simulink model "window_discriminator_5_2016"  (Simulink 8.8)
settings: Solver=FixedStepAuto  StartTime=0.0  StopTime=197  RelTol=1e-3
model workspace (MAT data in the model file):
  dac_stop_max = 3
  threshold = [-50; -300]
  win_start = [0; 0]
  win_stop = [3; 3]
PreLoadFcn:
  | load('DAC_data_0.mat')
libraries: simulink x28, dspswit3 x2
settings Model: SuppressorTable=22 serialization::archive 11 0 6 0 0 0 0 0  LogicAnalyzerGraphicalSettings="{\"cursors\":{\"activeCursor\":3,\"lockedCursors\":[],\"startingCursor\":0,\"times\":[0,4.8,0.93912000000000018,0.71536000000000011]},\"global\":{\"color\":\"#ff0000\",\"radix\":\"binary\",\"spacing\":20},\"panels\":{\"height\":100,\"startingTrace\":0,\"traces\":[{\"signalId\":\"f8938369-8c5b-4d01-b24d-9cd3e4e46d98\",\"type\":\"wave\"},{\"signalId\":\"94a143c0-ec74-472f-a084-edb62442a186\",\"type\":\"wave\"},{\"signalId\":\"701b10aa-339e-45e1-9be0-5d4a727281ed\",\"type\":\"wave\"},{\"signalId\":\"013b7378-a8ba-49d0-af91-3fbd95361aac\",\"type\":\"wave\"},{\"signalId\":\"480a99f9-8d02-4e3a-b326-8ef0fd120828\",\"type\":\"wave\"},{\"signalId\":\"c0ccc7cd-eb1d-43ab-8d7f-fc260d9b67b0\",\"type\":\"wave\"},{\"signalId\":\"28e0c295-4c7e-4ad9-b928-034bfdabfe57\",\"type\":\"wave\"},{\"signalId\":\"c5377225-ef61-4e55-bb70-795e7293a3ed\",\"type\":\"wave\"},{\"signalId\":\"41701cb5-c102-4d46-8782-f91045dab3d0\",\"type\":\"wave\"},{\"signalId\":\"59c9867a-a6c4-4660-9624-649cf34ef1b0\",\"type\":\"wave\"}],\"yOffset\":0},\"timeAxis\":{\"pixelsPerSecond\":1.8481561822124021E+6},\"trigger\":{\"enabled\":false,\"mode\":\"once\",\"samples\":200,\"signals\":{},\"stages\":{\"conditions\":[],\"operator\":\"AND\"}}}"  Creator=stefanobuccelli  LastModifiedBy=stefanobuccelli  SimulationMode=accelerator
settings DataIOCC: LimitDataPoints=off  SaveFormat=Dataset  SignalLoggingSaveFormat=Dataset
settings OptimizationCC: LifeSpan=auto
settings DebuggingCC: UnderspecifiedInitializationDetection=Simplified  MergeDetectMultiDrivingBlocksExec=error  FcnCallInpInsideContextMsg=error  StateNameClashWarn=none  SFUnexpectedBacktrackingDiag=error  SFNoUnconditionalDefaultTransitionDiag=error  SFExecutionAtInitializationDiag=warning
settings HardwareCC: ProdBitPerPointer=64  ProdBitPerSizeT=64  ProdBitPerPtrDiffT=64  ProdLargestAtomicFloat=Float  ProdIntDivRoundTo=Zero  ProdEndianess=LittleEndian  ProdWordSize=64  ProdHWDeviceType=Intel->x86-64 (Windows64)
settings ModelReferenceCC: PropagateSignalLabelsOutOfModel=on
settings GRTTargetCC: TargetLangStandard=C99 (ISO)  GeneratePreprocessorConditionals=Use local settings  CombineOutputUpdateFcns=on  GRTInterface=off
settings ConfigComp: CovMetricSettings=dwe  CovHtmlReporting=off  CovSaveCumulativeToWorkspaceVar=off  CovSaveSingleToWorkspaceVar=off  CovExternalEMLEnable=on

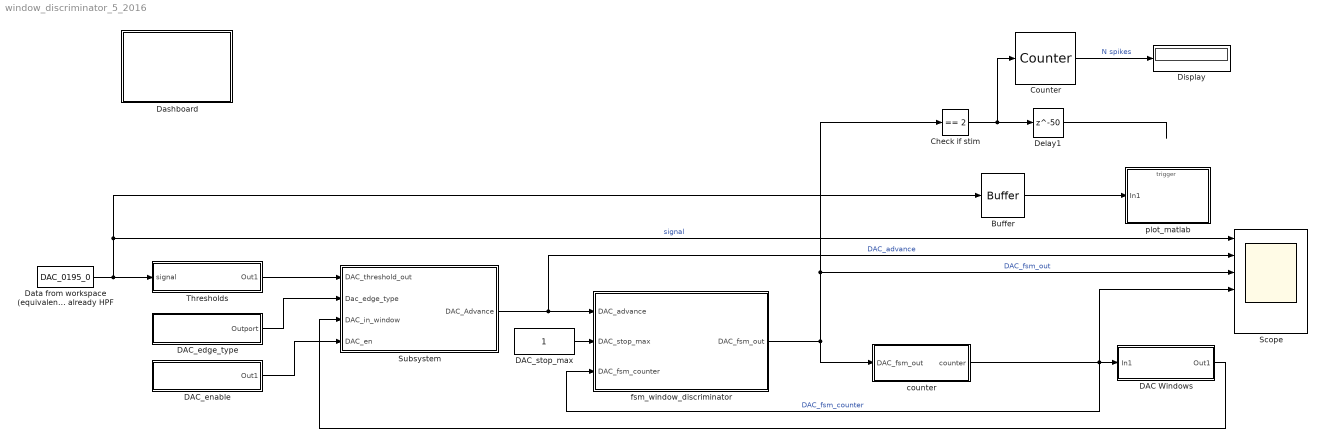
== system window_discriminator_5_2016 ==
  Buffer : Buffer  N=100  V=99  OutputFrames=off
  Check if stim : simulink/Logic and Bit Operations/Compare To Constant  relop===  const=2  OutDataTypeStr=boolean
  Counter : dspswit3/Counter  Direction=Up  CountEvent=Rising edge  CounterSize=User defined  MaxCount=1e6  InitialCount=0  Output=Count  HitValue=32  ResetInput=off  SamplesPerFrame=1  Ts=1  CntDtype=double  HitDtype=Logical
  DAC Windows : Subsystem
  DAC_edge_type : Subsystem
  DAC_enable : Subsystem
  DAC_stop_max : Constant  OutDataTypeStr=double
  Dashboard : Subsystem
  Data from workspace (equivalent  to the board_DAC_data the one already HPF : FromWorkspace  VariableName=DAC_0195_0  SampleTime=1/30000
  Delay1 : Delay  DelayLength=50
  Display : Display
  Scope : Scope  NumInputPorts=6
  Subsystem : Subsystem
  Thresholds : Subsystem
  counter : Subsystem
  fsm_window_discriminator : Stateflow chart  TreatAsAtomicUnit=on
  plot_matlab : Subsystem
  wires:
  fsm_window_discriminator/1(DAC_fsm_out) -> counter/1(DAC_fsm_out), Check if stim/1, Scope/3  "DAC_fsm_out"
  Data from workspace (equivalent  to the board_DAC_data the one already HPF/1 -> Buffer/1, Scope/1, Thresholds/1(signal)  "signal"
  Subsystem/1(DAC_Advance) -> Scope/2, fsm_window_discriminator/1(DAC_advance)  "DAC_advance"
  DAC_edge_type/1(Outport) -> Subsystem/2(Dac_edge_type)
  DAC_stop_max/1 -> fsm_window_discriminator/2(DAC_stop_max)
  Check if stim/1 -> Counter/1, Delay1/1
  Buffer/1 -> plot_matlab/1(In1)
  Delay1/1 -> ?
  DAC Windows/1(Out1) -> Subsystem/3(DAC_in_window)
  Thresholds/1(Out1) -> Subsystem/1(DAC_threshold_out)
  DAC_enable/1(Out1) -> Subsystem/4(DAC_en)
  counter/1(counter) -> fsm_window_discriminator/3(DAC_fsm_counter), DAC Windows/1(In1), Scope/4  "DAC_fsm_counter"
  Counter/1 -> Display/1  "N spikes"

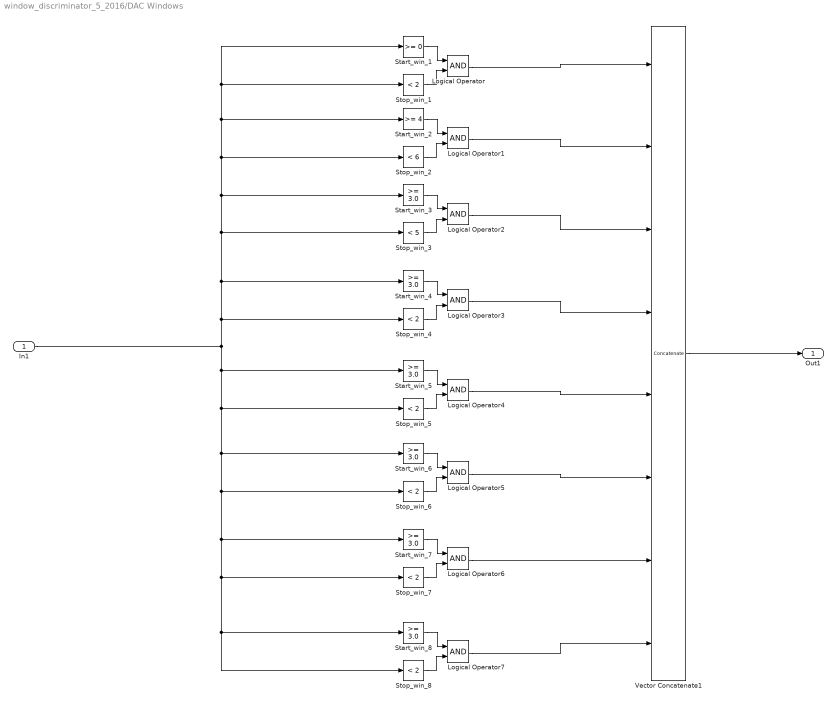
== system window_discriminator_5_2016/DAC Windows ==
  In1 : Inport
  Logical Operator{,1..7} (8 alike) : Logic  AllPortsSameDT=off  OutDataTypeStr=boolean
  Start_win_1 : simulink/Logic and Bit Operations/Compare To Constant  relop=>=  const=0  OutDataTypeStr=boolean
  Start_win_2 : simulink/Logic and Bit Operations/Compare To Constant  relop=>=  const=4  OutDataTypeStr=boolean
  Start_win_{3..8} (6 alike) : simulink/Logic and Bit Operations/Compare To Constant  relop=>=  const=3.0  OutDataTypeStr=boolean
  Stop_win_{1,4..8} (6 alike) : simulink/Logic and Bit Operations/Compare To Constant  relop=<  const=2  OutDataTypeStr=boolean
  Stop_win_2 : simulink/Logic and Bit Operations/Compare To Constant  relop=<  const=6  OutDataTypeStr=boolean
  Stop_win_3 : simulink/Logic and Bit Operations/Compare To Constant  relop=<  const=5  OutDataTypeStr=boolean
  Vector Concatenate1 : Concatenate  NumInputs=8
  Out1 : Outport
  wires:
  Vector Concatenate1/1 -> Out1/1
  Stop_win_1/1 -> Logical Operator/2
  Start_win_1/1 -> Logical Operator/1
  Logical Operator/1 -> Vector Concatenate1/1
  Logical Operator1/1 -> Vector Concatenate1/2
  Stop_win_2/1 -> Logical Operator1/2
  Start_win_2/1 -> Logical Operator1/1
  Stop_win_3/1 -> Logical Operator2/2
  Start_win_3/1 -> Logical Operator2/1
  Logical Operator2/1 -> Vector Concatenate1/3
  Start_win_4/1 -> Logical Operator3/1
  Stop_win_4/1 -> Logical Operator3/2
  Logical Operator3/1 -> Vector Concatenate1/4
  Stop_win_5/1 -> Logical Operator4/2
  Start_win_5/1 -> Logical Operator4/1
  Logical Operator4/1 -> Vector Concatenate1/5
  Start_win_6/1 -> Logical Operator5/1
  Logical Operator5/1 -> Vector Concatenate1/6
  Stop_win_6/1 -> Logical Operator5/2
  Stop_win_7/1 -> Logical Operator6/2
  Start_win_7/1 -> Logical Operator6/1
  Logical Operator6/1 -> Vector Concatenate1/7
  Stop_win_8/1 -> Logical Operator7/2
  Start_win_8/1 -> Logical Operator7/1
  Logical Operator7/1 -> Vector Concatenate1/8
  In1/1 -> Stop_win_5/1, Start_win_6/1, Stop_win_6/1, Start_win_7/1, Stop_win_7/1, Start_win_8/1, Stop_win_8/1, Start_win_5/1, Stop_win_4/1, Start_win_4/1, Stop_win_3/1, Start_win_3/1, Stop_win_2/1, Start_win_2/1, Stop_win_1/1, Start_win_1/1

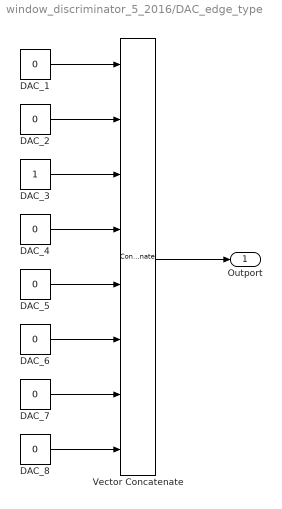
== system window_discriminator_5_2016/DAC_edge_type ==
  DAC_{1..2,4..8} (7 alike) : Constant  Value=0
  DAC_3 : Constant
  Vector Concatenate : Concatenate  NumInputs=8
  Outport : Outport
  wires:
  DAC_7/1 -> Vector Concatenate/7
  DAC_6/1 -> Vector Concatenate/6
  DAC_1/1 -> Vector Concatenate/1
  Vector Concatenate/1 -> Outport/1
  DAC_5/1 -> Vector Concatenate/5
  DAC_8/1 -> Vector Concatenate/8
  DAC_4/1 -> Vector Concatenate/4
  DAC_3/1 -> Vector Concatenate/3
  DAC_2/1 -> Vector Concatenate/2

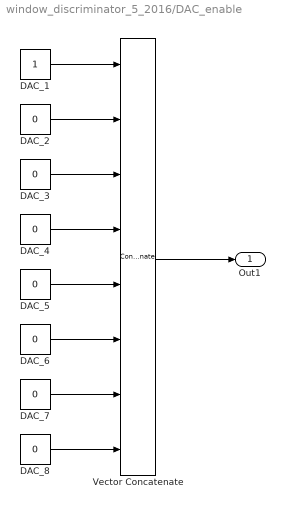
== system window_discriminator_5_2016/DAC_enable ==
  DAC_1 : Constant
  DAC_{2..8} (7 alike) : Constant  Value=0
  Vector Concatenate : Concatenate  NumInputs=8
  Out1 : Outport
  wires:
  DAC_1/1 -> Vector Concatenate/1
  DAC_4/1 -> Vector Concatenate/4
  DAC_2/1 -> Vector Concatenate/2
  DAC_8/1 -> Vector Concatenate/8
  Vector Concatenate/1 -> Out1/1
  DAC_3/1 -> Vector Concatenate/3
  DAC_7/1 -> Vector Concatenate/7
  DAC_5/1 -> Vector Concatenate/5
  DAC_6/1 -> Vector Concatenate/6

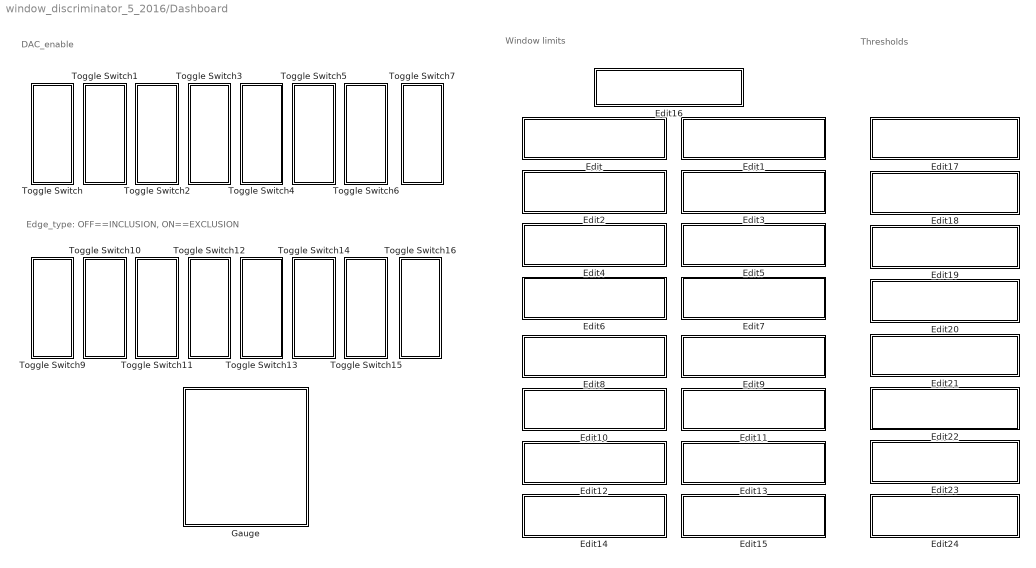
== system window_discriminator_5_2016/Dashboard ==
  note: Thresholds
  note: Window limits
  note: Edge_type: OFF==INCLUSION, ON==EXCLUSION
  note: DAC_enable
  Edit : Subsystem  Description=Replaced Block  mask(Replaced Block){}
      mask help: This block has been replaced with an empty subsystem because it used functionality that is unavailable in Simulink R2016b.
      mask Display: fprintf('Replaced: %s\n','Dashboard Widget')
  Edit1 : Subsystem  Description=Replaced Block  mask(Replaced Block){}
      mask help: This block has been replaced with an empty subsystem because it used functionality that is unavailable in Simulink R2016b.
      mask Display: fprintf('Replaced: %s\n','Dashboard Widget')
  Edit10 : Subsystem  Description=Replaced Block  mask(Replaced Block){}
      mask help: This block has been replaced with an empty subsystem because it used functionality that is unavailable in Simulink R2016b.
      mask Display: fprintf('Replaced: %s\n','Dashboard Widget')
  Edit11 : Subsystem  Description=Replaced Block  mask(Replaced Block){}
      mask help: This block has been replaced with an empty subsystem because it used functionality that is unavailable in Simulink R2016b.
      mask Display: fprintf('Replaced: %s\n','Dashboard Widget')
  Edit12 : Subsystem  Description=Replaced Block  mask(Replaced Block){}
      mask help: This block has been replaced with an empty subsystem because it used functionality that is unavailable in Simulink R2016b.
      mask Display: fprintf('Replaced: %s\n','Dashboard Widget')
  Edit13 : Subsystem  Description=Replaced Block  mask(Replaced Block){}
      mask help: This block has been replaced with an empty subsystem because it used functionality that is unavailable in Simulink R2016b.
      mask Display: fprintf('Replaced: %s\n','Dashboard Widget')
  Edit14 : Subsystem  Description=Replaced Block  mask(Replaced Block){}
      mask help: This block has been replaced with an empty subsystem because it used functionality that is unavailable in Simulink R2016b.
      mask Display: fprintf('Replaced: %s\n','Dashboard Widget')
  Edit15 : Subsystem  Description=Replaced Block  mask(Replaced Block){}
      mask help: This block has been replaced with an empty subsystem because it used functionality that is unavailable in Simulink R2016b.
      mask Display: fprintf('Replaced: %s\n','Dashboard Widget')
  Edit16 : Subsystem  Description=Replaced Block  mask(Replaced Block){}
      mask help: This block has been replaced with an empty subsystem because it used functionality that is unavailable in Simulink R2016b.
      mask Display: fprintf('Replaced: %s\n','Dashboard Widget')
  Edit17 : Subsystem  Description=Replaced Block  mask(Replaced Block){}
      mask help: This block has been replaced with an empty subsystem because it used functionality that is unavailable in Simulink R2016b.
      mask Display: fprintf('Replaced: %s\n','Dashboard Widget')
  Edit18 : Subsystem  Description=Replaced Block  mask(Replaced Block){}
      mask help: This block has been replaced with an empty subsystem because it used functionality that is unavailable in Simulink R2016b.
      mask Display: fprintf('Replaced: %s\n','Dashboard Widget')
  Edit19 : Subsystem  Description=Replaced Block  mask(Replaced Block){}
      mask help: This block has been replaced with an empty subsystem because it used functionality that is unavailable in Simulink R2016b.
      mask Display: fprintf('Replaced: %s\n','Dashboard Widget')
  Edit2 : Subsystem  Description=Replaced Block  mask(Replaced Block){}
      mask help: This block has been replaced with an empty subsystem because it used functionality that is unavailable in Simulink R2016b.
      mask Display: fprintf('Replaced: %s\n','Dashboard Widget')
  Edit20 : Subsystem  Description=Replaced Block  mask(Replaced Block){}
      mask help: This block has been replaced with an empty subsystem because it used functionality that is unavailable in Simulink R2016b.
      mask Display: fprintf('Replaced: %s\n','Dashboard Widget')
  Edit21 : Subsystem  Description=Replaced Block  mask(Replaced Block){}
      mask help: This block has been replaced with an empty subsystem because it used functionality that is unavailable in Simulink R2016b.
      mask Display: fprintf('Replaced: %s\n','Dashboard Widget')
  Edit22 : Subsystem  Description=Replaced Block  mask(Replaced Block){}
      mask help: This block has been replaced with an empty subsystem because it used functionality that is unavailable in Simulink R2016b.
      mask Display: fprintf('Replaced: %s\n','Dashboard Widget')
  Edit23 : Subsystem  Description=Replaced Block  mask(Replaced Block){}
      mask help: This block has been replaced with an empty subsystem because it used functionality that is unavailable in Simulink R2016b.
      mask Display: fprintf('Replaced: %s\n','Dashboard Widget')
  Edit24 : Subsystem  Description=Replaced Block  mask(Replaced Block){}
      mask help: This block has been replaced with an empty subsystem because it used functionality that is unavailable in Simulink R2016b.
      mask Display: fprintf('Replaced: %s\n','Dashboard Widget')
  Edit3 : Subsystem  Description=Replaced Block  mask(Replaced Block){}
      mask help: This block has been replaced with an empty subsystem because it used functionality that is unavailable in Simulink R2016b.
      mask Display: fprintf('Replaced: %s\n','Dashboard Widget')
  Edit4 : Subsystem  Description=Replaced Block  mask(Replaced Block){}
      mask help: This block has been replaced with an empty subsystem because it used functionality that is unavailable in Simulink R2016b.
      mask Display: fprintf('Replaced: %s\n','Dashboard Widget')
  Edit5 : Subsystem  Description=Replaced Block  mask(Replaced Block){}
      mask help: This block has been replaced with an empty subsystem because it used functionality that is unavailable in Simulink R2016b.
      mask Display: fprintf('Replaced: %s\n','Dashboard Widget')
  Edit6 : Subsystem  Description=Replaced Block  mask(Replaced Block){}
      mask help: This block has been replaced with an empty subsystem because it used functionality that is unavailable in Simulink R2016b.
      mask Display: fprintf('Replaced: %s\n','Dashboard Widget')
  Edit7 : Subsystem  Description=Replaced Block  mask(Replaced Block){}
      mask help: This block has been replaced with an empty subsystem because it used functionality that is unavailable in Simulink R2016b.
      mask Display: fprintf('Replaced: %s\n','Dashboard Widget')
  Edit8 : Subsystem  Description=Replaced Block  mask(Replaced Block){}
      mask help: This block has been replaced with an empty subsystem because it used functionality that is unavailable in Simulink R2016b.
      mask Display: fprintf('Replaced: %s\n','Dashboard Widget')
  Edit9 : Subsystem  Description=Replaced Block  mask(Replaced Block){}
      mask help: This block has been replaced with an empty subsystem because it used functionality that is unavailable in Simulink R2016b.
      mask Display: fprintf('Replaced: %s\n','Dashboard Widget')
  Gauge : Subsystem  DialogController=hmiCreateDDGDialog  DialogControllerArgs=DataTag1  IsWebBlock=on  mask(MWDashboardBlock){webBlockId=9508d0a0-9094-44a2-b73a-dcd38a83431a, webBlockType=circulargauge, ShowInLibBrowser=on, ShowInitialText=on, HMISrcModelName=[]}
      mask prompts: webBlockId "WebBlock Id"; webBlockType "WebBlock Type"; HMISrcModelName "Source Model"
      mask help: SimulinkHMI:dialogs:CircularGaugeDialogDesc
      mask Help: helpview([docroot '/mapfiles/simulink.map'], 'hmi_gauge')
      mask Display:
      | if strcmp(get_param(bdroot(gcb),'BlockDiagramType'), 'library')
      |     image([(matlabroot) '/toolbox/simulink/hmi/icons/CircularGauge.png']);
      | end
  Toggle Switch : Subsystem  DialogController=hmiCreateDDGDialog  DialogControllerArgs=DataTag2  IsWebBlock=on  mask(MWDashboardBlock){webBlockId=a4df6f67-033a-4993-a7c4-946ed6eae349, webBlockType=toggleswitch, ShowInLibBrowser=on, ShowInitialText=on, HMISrcModelName=window_discriminator_5_2016}
      mask prompts: webBlockId "WebBlock Id"; webBlockType "WebBlock Type"; HMISrcModelName "Source Model"
      mask help: Set on/off value to tune parameters or variables.
      mask Help: helpview([docroot '/mapfiles/simulink.map'], 'hmi_switch')
      mask Display:
      | if strcmp(get_param(bdroot(gcb),'BlockDiagramType'),'library')
      |  image([(matlabroot) '/toolbox/simulink/hmi/icons/ToggleSwitch.png'])
      | end
  Toggle Switch1 : Subsystem  DialogController=hmiCreateDDGDialog  DialogControllerArgs=DataTag3  IsWebBlock=on  mask(MWDashboardBlock){webBlockId=e7fd446b-ef83-4929-84a5-122acd6de0d1, webBlockType=toggleswitch, ShowInLibBrowser=on, ShowInitialText=on, HMISrcModelName=window_discriminator_5_2016}
      mask prompts: webBlockId "WebBlock Id"; webBlockType "WebBlock Type"; HMISrcModelName "Source Model"
      mask help: Set on/off value to tune parameters or variables.
      mask Help: helpview([docroot '/mapfiles/simulink.map'], 'hmi_switch')
      mask Display:
      | if strcmp(get_param(bdroot(gcb),'BlockDiagramType'),'library')
      |  image([(matlabroot) '/toolbox/simulink/hmi/icons/ToggleSwitch.png'])
      | end
  Toggle Switch10 : Subsystem  DialogController=hmiCreateDDGDialog  DialogControllerArgs=DataTag4  IsWebBlock=on  mask(MWDashboardBlock){webBlockId=a65b6b20-e6e8-4e80-9491-7171f8859a10, webBlockType=toggleswitch, ShowInLibBrowser=on, ShowInitialText=on, HMISrcModelName=window_discriminator_5_2016}
      mask prompts: webBlockId "WebBlock Id"; webBlockType "WebBlock Type"; HMISrcModelName "Source Model"
      mask help: Set on/off value to tune parameters or variables.
      mask Help: helpview([docroot '/mapfiles/simulink.map'], 'hmi_switch')
      mask Display:
      | if strcmp(get_param(bdroot(gcb),'BlockDiagramType'),'library')
      |  image([(matlabroot) '/toolbox/simulink/hmi/icons/ToggleSwitch.png'])
      | end
  Toggle Switch11 : Subsystem  DialogController=hmiCreateDDGDialog  DialogControllerArgs=DataTag5  IsWebBlock=on  mask(MWDashboardBlock){webBlockId=fbce3a53-e423-4e67-acb0-0b77f95405cc, webBlockType=toggleswitch, ShowInLibBrowser=on, ShowInitialText=on, HMISrcModelName=window_discriminator_5_2016}
      mask prompts: webBlockId "WebBlock Id"; webBlockType "WebBlock Type"; HMISrcModelName "Source Model"
      mask help: Set on/off value to tune parameters or variables.
      mask Help: helpview([docroot '/mapfiles/simulink.map'], 'hmi_switch')
      mask Display:
      | if strcmp(get_param(bdroot(gcb),'BlockDiagramType'),'library')
      |  image([(matlabroot) '/toolbox/simulink/hmi/icons/ToggleSwitch.png'])
      | end
  Toggle Switch12 : Subsystem  DialogController=hmiCreateDDGDialog  DialogControllerArgs=DataTag6  IsWebBlock=on  mask(MWDashboardBlock){webBlockId=6d69be38-9978-4d4e-95df-5f6f10c8cd42, webBlockType=toggleswitch, ShowInLibBrowser=on, ShowInitialText=on, HMISrcModelName=window_discriminator_5_2016}
      mask prompts: webBlockId "WebBlock Id"; webBlockType "WebBlock Type"; HMISrcModelName "Source Model"
      mask help: Set on/off value to tune parameters or variables.
      mask Help: helpview([docroot '/mapfiles/simulink.map'], 'hmi_switch')
      mask Display:
      | if strcmp(get_param(bdroot(gcb),'BlockDiagramType'),'library')
      |  image([(matlabroot) '/toolbox/simulink/hmi/icons/ToggleSwitch.png'])
      | end
  Toggle Switch13 : Subsystem  DialogController=hmiCreateDDGDialog  DialogControllerArgs=DataTag7  IsWebBlock=on  mask(MWDashboardBlock){webBlockId=e1fd5474-c792-436d-8149-89277fa4e19b, webBlockType=toggleswitch, ShowInLibBrowser=on, ShowInitialText=on, HMISrcModelName=window_discriminator_5_2016}
      mask prompts: webBlockId "WebBlock Id"; webBlockType "WebBlock Type"; HMISrcModelName "Source Model"
      mask help: Set on/off value to tune parameters or variables.
      mask Help: helpview([docroot '/mapfiles/simulink.map'], 'hmi_switch')
      mask Display:
      | if strcmp(get_param(bdroot(gcb),'BlockDiagramType'),'library')
      |  image([(matlabroot) '/toolbox/simulink/hmi/icons/ToggleSwitch.png'])
      | end
  Toggle Switch14 : Subsystem  DialogController=hmiCreateDDGDialog  DialogControllerArgs=DataTag8  IsWebBlock=on  mask(MWDashboardBlock){webBlockId=ebe499df-f77e-4a00-b3f5-a27d082e09c1, webBlockType=toggleswitch, ShowInLibBrowser=on, ShowInitialText=on, HMISrcModelName=window_discriminator_5_2016}
      mask prompts: webBlockId "WebBlock Id"; webBlockType "WebBlock Type"; HMISrcModelName "Source Model"
      mask help: Set on/off value to tune parameters or variables.
      mask Help: helpview([docroot '/mapfiles/simulink.map'], 'hmi_switch')
      mask Display:
      | if strcmp(get_param(bdroot(gcb),'BlockDiagramType'),'library')
      |  image([(matlabroot) '/toolbox/simulink/hmi/icons/ToggleSwitch.png'])
      | end
  Toggle Switch15 : Subsystem  DialogController=hmiCreateDDGDialog  DialogControllerArgs=DataTag9  IsWebBlock=on  mask(MWDashboardBlock){webBlockId=d267d004-1aa6-44bb-ac36-4a6fc3ab3b76, webBlockType=toggleswitch, ShowInLibBrowser=on, ShowInitialText=on, HMISrcModelName=window_discriminator_5_2016}
      mask prompts: webBlockId "WebBlock Id"; webBlockType "WebBlock Type"; HMISrcModelName "Source Model"
      mask help: Set on/off value to tune parameters or variables.
      mask Help: helpview([docroot '/mapfiles/simulink.map'], 'hmi_switch')
      mask Display:
      | if strcmp(get_param(bdroot(gcb),'BlockDiagramType'),'library')
      |  image([(matlabroot) '/toolbox/simulink/hmi/icons/ToggleSwitch.png'])
      | end
  Toggle Switch16 : Subsystem  DialogController=hmiCreateDDGDialog  DialogControllerArgs=DataTag10  IsWebBlock=on  mask(MWDashboardBlock){webBlockId=55743ebe-cd36-47aa-963c-6ddae4fb2fee, webBlockType=toggleswitch, ShowInLibBrowser=on, ShowInitialText=on, HMISrcModelName=window_discriminator_5_2016}
      mask prompts: webBlockId "WebBlock Id"; webBlockType "WebBlock Type"; HMISrcModelName "Source Model"
      mask help: Set on/off value to tune parameters or variables.
      mask Help: helpview([docroot '/mapfiles/simulink.map'], 'hmi_switch')
      mask Display:
      | if strcmp(get_param(bdroot(gcb),'BlockDiagramType'),'library')
      |  image([(matlabroot) '/toolbox/simulink/hmi/icons/ToggleSwitch.png'])
      | end
  Toggle Switch2 : Subsystem  DialogController=hmiCreateDDGDialog  DialogControllerArgs=DataTag11  IsWebBlock=on  mask(MWDashboardBlock){webBlockId=a27b2da1-d5a2-4f2a-b110-d4112ff455c2, webBlockType=toggleswitch, ShowInLibBrowser=on, ShowInitialText=on, HMISrcModelName=window_discriminator_5_2016}
      mask prompts: webBlockId "WebBlock Id"; webBlockType "WebBlock Type"; HMISrcModelName "Source Model"
      mask help: Set on/off value to tune parameters or variables.
      mask Help: helpview([docroot '/mapfiles/simulink.map'], 'hmi_switch')
      mask Display:
      | if strcmp(get_param(bdroot(gcb),'BlockDiagramType'),'library')
      |  image([(matlabroot) '/toolbox/simulink/hmi/icons/ToggleSwitch.png'])
      | end
  Toggle Switch3 : Subsystem  DialogController=hmiCreateDDGDialog  DialogControllerArgs=DataTag12  IsWebBlock=on  mask(MWDashboardBlock){webBlockId=1aa30ff8-90ff-4a5e-b5b8-f3415d0db09d, webBlockType=toggleswitch, ShowInLibBrowser=on, ShowInitialText=on, HMISrcModelName=window_discriminator_5_2016}
      mask prompts: webBlockId "WebBlock Id"; webBlockType "WebBlock Type"; HMISrcModelName "Source Model"
      mask help: Set on/off value to tune parameters or variables.
      mask Help: helpview([docroot '/mapfiles/simulink.map'], 'hmi_switch')
      mask Display:
      | if strcmp(get_param(bdroot(gcb),'BlockDiagramType'),'library')
      |  image([(matlabroot) '/toolbox/simulink/hmi/icons/ToggleSwitch.png'])
      | end
  Toggle Switch4 : Subsystem  DialogController=hmiCreateDDGDialog  DialogControllerArgs=DataTag13  IsWebBlock=on  mask(MWDashboardBlock){webBlockId=f9d11862-86b7-40df-9d66-ca6db8f8b2a5, webBlockType=toggleswitch, ShowInLibBrowser=on, ShowInitialText=on, HMISrcModelName=window_discriminator_5_2016}
      mask prompts: webBlockId "WebBlock Id"; webBlockType "WebBlock Type"; HMISrcModelName "Source Model"
      mask help: Set on/off value to tune parameters or variables.
      mask Help: helpview([docroot '/mapfiles/simulink.map'], 'hmi_switch')
      mask Display:
      | if strcmp(get_param(bdroot(gcb),'BlockDiagramType'),'library')
      |  image([(matlabroot) '/toolbox/simulink/hmi/icons/ToggleSwitch.png'])
      | end
  Toggle Switch5 : Subsystem  DialogController=hmiCreateDDGDialog  DialogControllerArgs=DataTag14  IsWebBlock=on  mask(MWDashboardBlock){webBlockId=ea86c505-88e3-44bc-89e9-800f836199b1, webBlockType=toggleswitch, ShowInLibBrowser=on, ShowInitialText=on, HMISrcModelName=window_discriminator_5_2016}
      mask prompts: webBlockId "WebBlock Id"; webBlockType "WebBlock Type"; HMISrcModelName "Source Model"
      mask help: Set on/off value to tune parameters or variables.
      mask Help: helpview([docroot '/mapfiles/simulink.map'], 'hmi_switch')
      mask Display:
      | if strcmp(get_param(bdroot(gcb),'BlockDiagramType'),'library')
      |  image([(matlabroot) '/toolbox/simulink/hmi/icons/ToggleSwitch.png'])
      | end
  Toggle Switch6 : Subsystem  DialogController=hmiCreateDDGDialog  DialogControllerArgs=DataTag15  IsWebBlock=on  mask(MWDashboardBlock){webBlockId=f085ddb9-8199-42f6-aabb-5ef1fa30c03a, webBlockType=toggleswitch, ShowInLibBrowser=on, ShowInitialText=on, HMISrcModelName=window_discriminator_5_2016}
      mask prompts: webBlockId "WebBlock Id"; webBlockType "WebBlock Type"; HMISrcModelName "Source Model"
      mask help: Set on/off value to tune parameters or variables.
      mask Help: helpview([docroot '/mapfiles/simulink.map'], 'hmi_switch')
      mask Display:
      | if strcmp(get_param(bdroot(gcb),'BlockDiagramType'),'library')
      |  image([(matlabroot) '/toolbox/simulink/hmi/icons/ToggleSwitch.png'])
      | end
  Toggle Switch7 : Subsystem  DialogController=hmiCreateDDGDialog  DialogControllerArgs=DataTag16  IsWebBlock=on  mask(MWDashboardBlock){webBlockId=fc189f06-1e95-4706-80b4-9c62c07b2b89, webBlockType=toggleswitch, ShowInLibBrowser=on, ShowInitialText=on, HMISrcModelName=window_discriminator_5_2016}
      mask prompts: webBlockId "WebBlock Id"; webBlockType "WebBlock Type"; HMISrcModelName "Source Model"
      mask help: Set on/off value to tune parameters or variables.
      mask Help: helpview([docroot '/mapfiles/simulink.map'], 'hmi_switch')
      mask Display:
      | if strcmp(get_param(bdroot(gcb),'BlockDiagramType'),'library')
      |  image([(matlabroot) '/toolbox/simulink/hmi/icons/ToggleSwitch.png'])
      | end
  Toggle Switch9 : Subsystem  DialogController=hmiCreateDDGDialog  DialogControllerArgs=DataTag17  IsWebBlock=on  mask(MWDashboardBlock){webBlockId=6eb4bb6c-1295-41da-a201-0e4d216872f3, webBlockType=toggleswitch, ShowInLibBrowser=on, ShowInitialText=on, HMISrcModelName=window_discriminator_5_2016}
      mask prompts: webBlockId "WebBlock Id"; webBlockType "WebBlock Type"; HMISrcModelName "Source Model"
      mask help: Set on/off value to tune parameters or variables.
      mask Help: helpview([docroot '/mapfiles/simulink.map'], 'hmi_switch')
      mask Display:
      | if strcmp(get_param(bdroot(gcb),'BlockDiagramType'),'library')
      |  image([(matlabroot) '/toolbox/simulink/hmi/icons/ToggleSwitch.png'])
      | end

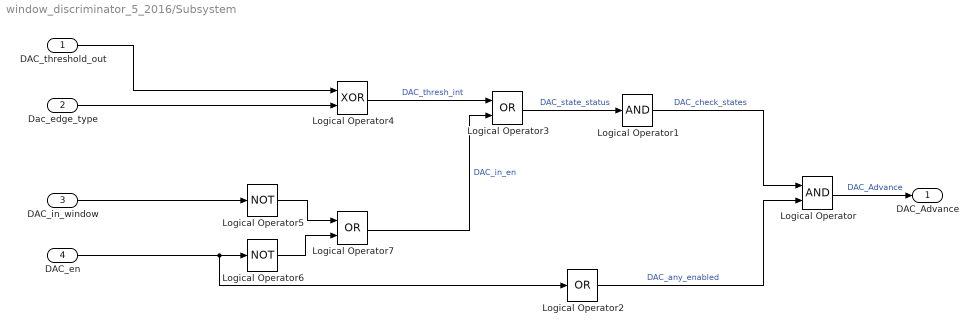
== system window_discriminator_5_2016/Subsystem ==
  DAC_threshold_out : Inport
  Dac_edge_type : Inport  Port=2
  DAC_in_window : Inport  Port=3
  DAC_en : Inport  Port=4
  Logical Operator : Logic  AllPortsSameDT=off  OutDataTypeStr=boolean
  Logical Operator1 : Logic  Inputs=1  AllPortsSameDT=off  OutDataTypeStr=boolean
  Logical Operator2 : Logic  Operator=OR  Inputs=1  AllPortsSameDT=off  OutDataTypeStr=boolean
  Logical Operator3 : Logic  Operator=OR  AllPortsSameDT=off  OutDataTypeStr=boolean
  Logical Operator4 : Logic  Operator=XOR  AllPortsSameDT=off  OutDataTypeStr=boolean
  Logical Operator5 : Logic  Operator=NOT  Inputs=1  AllPortsSameDT=off  OutDataTypeStr=boolean
  Logical Operator6 : Logic  Operator=NOT  Inputs=1  AllPortsSameDT=off  OutDataTypeStr=boolean
  Logical Operator7 : Logic  Operator=OR  AllPortsSameDT=off  OutDataTypeStr=boolean
  DAC_Advance : Outport
  wires:
  Logical Operator/1 -> DAC_Advance/1  "DAC_Advance"
  Logical Operator2/1 -> Logical Operator/2  "DAC_any_enabled"
  Logical Operator1/1 -> Logical Operator/1  "DAC_check_states"
  Logical Operator4/1 -> Logical Operator3/1  "DAC_thresh_int"
  Logical Operator5/1 -> Logical Operator7/1
  DAC_threshold_out/1 -> Logical Operator4/1
  DAC_en/1 -> Logical Operator2/1, Logical Operator6/1
  Logical Operator3/1 -> Logical Operator1/1  "DAC_state_status"
  Logical Operator6/1 -> Logical Operator7/2
  Logical Operator7/1 -> Logical Operator3/2  "DAC_in_en"
  Dac_edge_type/1 -> Logical Operator4/2
  DAC_in_window/1 -> Logical Operator5/1

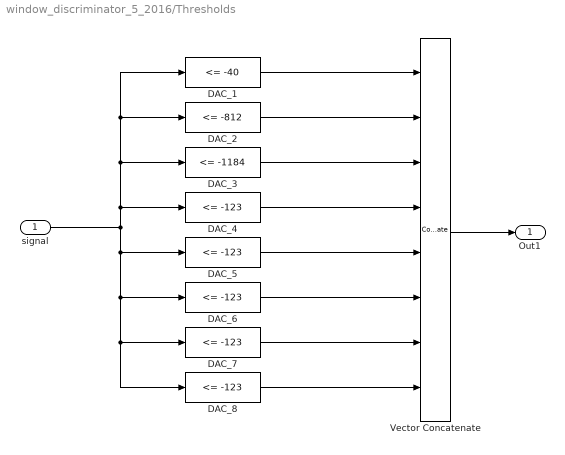
== system window_discriminator_5_2016/Thresholds ==
  signal : Inport
  DAC_1 : simulink/Logic and Bit Operations/Compare To Constant  relop=<=  const=-40  OutDataTypeStr=boolean
  DAC_2 : simulink/Logic and Bit Operations/Compare To Constant  relop=<=  const=-812  OutDataTypeStr=boolean
  DAC_3 : simulink/Logic and Bit Operations/Compare To Constant  relop=<=  const=-1184  OutDataTypeStr=boolean
  DAC_{4..8} (5 alike) : simulink/Logic and Bit Operations/Compare To Constant  relop=<=  const=-123  OutDataTypeStr=boolean
  Vector Concatenate : Concatenate  NumInputs=8
  Out1 : Outport
  wires:
  Vector Concatenate/1 -> Out1/1
  signal/1 -> DAC_8/1, DAC_7/1, DAC_6/1, DAC_5/1, DAC_4/1, DAC_3/1, DAC_2/1, DAC_1/1
  DAC_1/1 -> Vector Concatenate/1
  DAC_2/1 -> Vector Concatenate/2
  DAC_4/1 -> Vector Concatenate/4
  DAC_3/1 -> Vector Concatenate/3
  DAC_6/1 -> Vector Concatenate/6
  DAC_7/1 -> Vector Concatenate/7
  DAC_5/1 -> Vector Concatenate/5
  DAC_8/1 -> Vector Concatenate/8

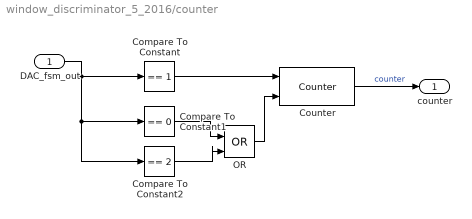
== system window_discriminator_5_2016/counter ==
  DAC_fsm_out : Inport
  Compare To Constant : simulink/Logic and Bit Operations/Compare To Constant  relop===  const=1  OutDataTypeStr=boolean
  Compare To Constant1 : simulink/Logic and Bit Operations/Compare To Constant  relop===  const=0  OutDataTypeStr=boolean
  Compare To Constant2 : simulink/Logic and Bit Operations/Compare To Constant  relop===  const=2  OutDataTypeStr=boolean
  Counter : dspswit3/Counter  Direction=Up  CountEvent=Non-zero sample  CounterSize=User defined  MaxCount=255  InitialCount=0  Output=Count  HitValue=32  ResetInput=on  SamplesPerFrame=1  Ts=1  CntDtype=double  HitDtype=Logical
  OR : Logic  Operator=OR  IconShape=distinctive  AllPortsSameDT=off  OutDataTypeStr=boolean
  counter : Outport
  wires:
  Counter/1 -> counter/1  "counter"
  Compare To Constant2/1 -> OR/2
  Compare To Constant/1 -> Counter/1
  Compare To Constant1/1 -> OR/1
  OR/1 -> Counter/2
  DAC_fsm_out/1 -> Compare To Constant2/1, Compare To Constant1/1, Compare To Constant/1

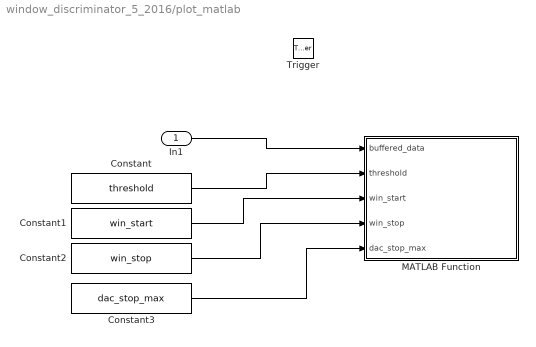
== system window_discriminator_5_2016/plot_matlab ==
  In1 : Inport
  Trigger : TriggerPort  VariantControl=Variant  PortDimensions=1
  Constant : Constant  Value=threshold
  Constant1 : Constant  Value=win_start
  Constant2 : Constant  Value=win_stop
  Constant3 : Constant  Value=dac_stop_max
  MATLAB Function : MATLAB Function  TreatAsAtomicUnit=on
  wires:
  In1/1 -> MATLAB Function/1(buffered_data)
  Constant1/1 -> MATLAB Function/3(win_start)
  Constant/1 -> MATLAB Function/2(threshold)
  Constant2/1 -> MATLAB Function/4(win_stop)
  Constant3/1 -> MATLAB Function/5(dac_stop_max)

== system window_discriminator_5_2016/Dashboard/Edit ==

== system window_discriminator_5_2016/Dashboard/Edit1 ==

== system window_discriminator_5_2016/Dashboard/Edit10 ==

== system window_discriminator_5_2016/Dashboard/Edit11 ==

== system window_discriminator_5_2016/Dashboard/Edit12 ==

== system window_discriminator_5_2016/Dashboard/Edit13 ==

== system window_discriminator_5_2016/Dashboard/Edit14 ==

== system window_discriminator_5_2016/Dashboard/Edit15 ==

== system window_discriminator_5_2016/Dashboard/Edit16 ==

== system window_discriminator_5_2016/Dashboard/Edit17 ==

== system window_discriminator_5_2016/Dashboard/Edit18 ==

== system window_discriminator_5_2016/Dashboard/Edit19 ==

== system window_discriminator_5_2016/Dashboard/Edit2 ==

== system window_discriminator_5_2016/Dashboard/Edit20 ==

== system window_discriminator_5_2016/Dashboard/Edit21 ==

== system window_discriminator_5_2016/Dashboard/Edit22 ==

== system window_discriminator_5_2016/Dashboard/Edit23 ==

== system window_discriminator_5_2016/Dashboard/Edit24 ==

== system window_discriminator_5_2016/Dashboard/Edit3 ==

== system window_discriminator_5_2016/Dashboard/Edit4 ==

== system window_discriminator_5_2016/Dashboard/Edit5 ==

== system window_discriminator_5_2016/Dashboard/Edit6 ==

== system window_discriminator_5_2016/Dashboard/Edit7 ==

== system window_discriminator_5_2016/Dashboard/Edit8 ==

== system window_discriminator_5_2016/Dashboard/Edit9 ==

== system window_discriminator_5_2016/Dashboard/Gauge ==

== system window_discriminator_5_2016/Dashboard/Toggle Switch ==

== system window_discriminator_5_2016/Dashboard/Toggle Switch1 ==

== system window_discriminator_5_2016/Dashboard/Toggle Switch10 ==

== system window_discriminator_5_2016/Dashboard/Toggle Switch11 ==

== system window_discriminator_5_2016/Dashboard/Toggle Switch12 ==

== system window_discriminator_5_2016/Dashboard/Toggle Switch13 ==

== system window_discriminator_5_2016/Dashboard/Toggle Switch14 ==

== system window_discriminator_5_2016/Dashboard/Toggle Switch15 ==

== system window_discriminator_5_2016/Dashboard/Toggle Switch16 ==

== system window_discriminator_5_2016/Dashboard/Toggle Switch2 ==

== system window_discriminator_5_2016/Dashboard/Toggle Switch3 ==

== system window_discriminator_5_2016/Dashboard/Toggle Switch4 ==

== system window_discriminator_5_2016/Dashboard/Toggle Switch5 ==

== system window_discriminator_5_2016/Dashboard/Toggle Switch6 ==

== system window_discriminator_5_2016/Dashboard/Toggle Switch7 ==

== system window_discriminator_5_2016/Dashboard/Toggle Switch9 ==

== matlab function plot_matlab/MATLAB Function ==
  data: buffered_data input double; threshold input double; win_start input double; win_stop input double; dac_stop_max input double
function  fcn(buffered_data,threshold,win_start,win_stop,dac_stop_max)
shift=length(buffered_data)/2;
figure(1)
plot((1:length(buffered_data))-shift,buffered_data,'k')
hold on
for curr_DAC=1:length(threshold)
    plot([win_start(curr_DAC):win_stop(curr_DAC)-1]-dac_stop_max,repmat(threshold(curr_DAC),1,length(win_start(curr_DAC):win_stop(curr_DAC)-1)),'b')
end
% the -1 in the start-stop win position is due to the delay (I guess XD)

== stateflow chart fsm_window_discriminator ==
  settings: stateMachineType=MOORE_MACHINE  executeAtInitialization=1
  state IDLE
    DAC_fsm_out=0
  state TRACK
    DAC_fsm_out=1
  state STIM
    DAC_fsm_out=2
  (default) -> IDLE
  STIM -> IDLE
  TRACK -> IDLE [order 2] : [~DAC_advance]
  IDLE -> TRACK : [DAC_advance]
  TRACK -> TRACK [order 3] : [DAC_fsm_counter~=DAC_stop_max]
  TRACK -> STIM [order 1] : [DAC_fsm_counter==DAC_stop_max]
  data: DAC_advance input double; DAC_fsm_out output double =0; DAC_stop_max input double; DAC_fsm_counter input double =0
